simulink model "LR_Traject_Sim"  (R2017b)
settings: Solver=ode4  StartTime=0  StopTime=100  FixedStep=0.05  RelTol=1e-7
model workspace (MAT data in the model file):
  Object = Simulink.LookupTable
  Object.Table = Simulink.lookuptable.Table
  Object.Table.Dimensions = [0 0]
  Object.Table.DataType = 'auto'
  Object.Table.FieldName = 'Table'
  Object.Breakpoints = Simulink.lookuptable.Breakpoint
  Object.Breakpoints.TunableSizeName = 'N1'
  Object.Breakpoints.Dimensions = [0 0]
  Object.Breakpoints.DataType = 'auto'
  Object.Breakpoints.FieldName = 'BP1'
  Object.SupportTunableSize = 0
  Object.StructTypeInfo = Simulink.lookuptable.StructTypeInfo
  Object.StructTypeInfo.DataScope = 'Auto'
undefined symbols (not defined in the file or in its folder): Conditions, Eng, Roc
settings Model: Creator=adamb  LastModifiedBy=dc0069
settings SolverCC: ZeroCrossAlgorithm=Adaptive
settings DataIOCC: SaveFormat=StructureWithTime
settings OptimizationCC: LifeSpan=inf
settings DebuggingCC: AlgebraicLoopMsg=none  ArtificialAlgebraicLoopMsg=none  SFExecutionAtInitializationDiag=none
settings HardwareCC: ProdBitPerSizeT=32  ProdBitPerPtrDiffT=32  ProdWordSize=32  ProdHWDeviceType=Specified
settings CodeAppCC: StateflowObjectComments=on
settings SimscapeCC: SimscapeNormalizeSystem=off
settings ConfigurationSet: Description=SimMechanics 2G

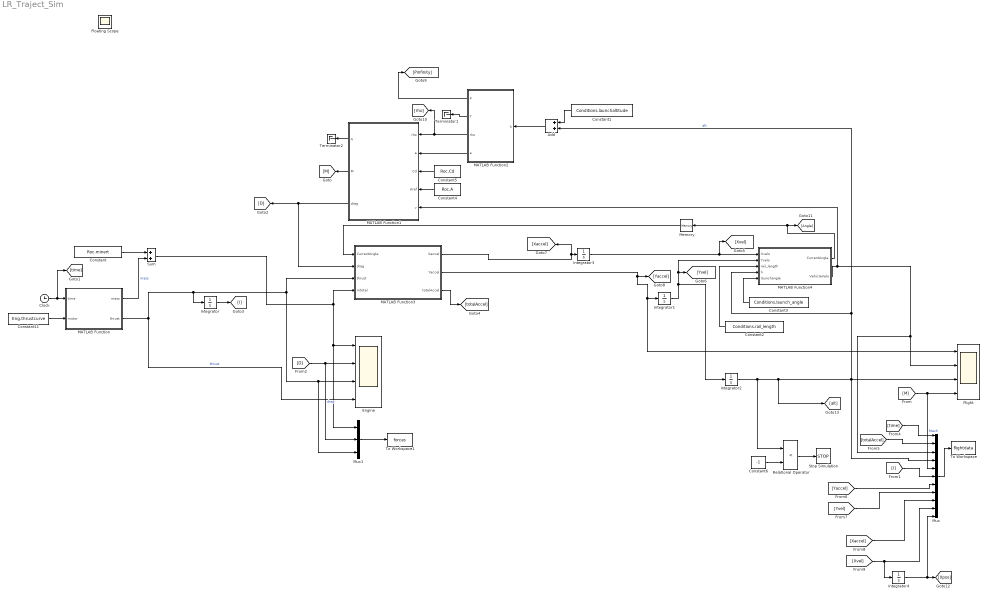
== system LR_Traject_Sim ==
  Add : Sum
  Clock : Clock
  Constant : Constant  Value=Roc.minert
  Constant1 : Constant  Value=Conditions.launchaltitude
  Constant11 : Constant  Value=Eng.thrustcurve
  Constant2 : Constant  Value=Conditions.rail_length
  Constant3 : Constant  Value=Conditions.launch_angle
  Constant4 : Constant  Value=Roc.A
  Constant5 : Constant  Value=Roc.Cd  VectorParams1D=off
  Constant6 : Constant  Value=-1
  Engine : Scope  NumInputPorts=4
  Flight : Scope  NumInputPorts=4
  Integrator{,1..4} (5 alike) : Integrator
  MATLAB Function : MATLAB Function  TreatAsAtomicUnit=on
  MATLAB Function1 : MATLAB Function  TreatAsAtomicUnit=on
  MATLAB Function2 : MATLAB Function  TreatAsAtomicUnit=on
  MATLAB Function3 : MATLAB Function  TreatAsAtomicUnit=on
  MATLAB Function4 : MATLAB Function  TreatAsAtomicUnit=on
  Memory : Memory
  Mux : Mux  Inputs=11
  Mux1 : Mux  Inputs=3
  Relational Operator : RelationalOperator  Operator=<  OutDataTypeStr=boolean  RndMeth=Nearest
  Stop Simulation : Stop
  Sum : Sum
  Terminator1 : Terminator
  Terminator2 : Terminator
  To Workspace : ToWorkspace  VariableName=flightdata  SampleTime=-1
  To Workspace1 : ToWorkspace  VariableName=forces  SampleTime=-1
  Floating Scope : Scope
  wires:
  MATLAB Function/1(mass) -> Sum/2  "mass"
  MATLAB Function/2(thrust) -> Engine/4, Mux1/3, Engine/3, MATLAB Function3/3(thrust), Integrator/1  "thrust"
  Integrator1/1 -> Integrator2/1, [Yvel], MATLAB Function4/2(Yvelo)
  Integrator2/1 -> Relational Operator/1, Add/2, MATLAB Function4/4(h), Flight/3, Mux/4, [alt]  "alt"
  Constant4/1 -> MATLAB Function1/4(Aref)
  Constant5/1 -> MATLAB Function1/3(Cd)
  MATLAB Function1/2(M) -> [M]
  [M] -> Mux/5, Flight/4  "Mach"
  MATLAB Function1/3(drag) -> [D], MATLAB Function3/2(drag)
  Relational Operator/1 -> Stop Simulation/1
  Constant6/1 -> Relational Operator/2
  MATLAB Function2/4(a) -> MATLAB Function1/2(a)
  MATLAB Function2/3(rho) -> [rho], MATLAB Function1/1(rho)
  Mux/1 -> To Workspace/1
  MATLAB Function2/2(T) -> Terminator1/1
  [D] -> Mux1/2, Engine/2  "drag"
  Mux1/1 -> To Workspace1/1
  MATLAB Function1/1(q) -> Terminator2/1
  MATLAB Function2/1(P) -> [Pinfinity]
  Clock/1 -> MATLAB Function/1(time), [time]
  [time] -> Mux/1
  MATLAB Function3/2(Yaccel) -> Flight/1, Integrator1/1, [Yaccel]
  Integrator3/1 -> [Xvel], MATLAB Function4/1(Xvelo)
  MATLAB Function4/2(VehicleVelo) -> MATLAB Function1/5(v), Flight/2, Mux/3
  Integrator/1 -> [I]
  [I] -> Mux/6
  Add/1 -> MATLAB Function2/1(h)
  Constant1/1 -> Add/1
  MATLAB Function4/1(CurrentAngle) -> [Angle], Memory/1
  Constant2/1 -> MATLAB Function4/3(rail_length)
  Constant3/1 -> MATLAB Function4/5(launchangle)
  Memory/1 -> MATLAB Function3/1(CurrentAngle)
  [totalAccel] -> Mux/2
  [Xaccel] -> Mux/9
  [Xvel] -> Integrator4/1, Mux/10
  [Yvel] -> Mux/8
  [Yaccel] -> Mux/7
  Integrator4/1 -> [Xpos], Mux/11
  MATLAB Function3/1(Xaccel) -> [Xaccel], Integrator3/1
  MATLAB Function3/3(totalAccel) -> [totalAccel]
  Constant/1 -> Sum/1
  Sum/1 -> Mux1/1, Engine/1, MATLAB Function3/4(mtotal)
  Constant11/1 -> MATLAB Function/2(motor)

== matlab function LR_Traject_Sim/MATLAB Function1 ==
  data: rho input; a input; q output; M output; Cd input; Aref input; v input; drag output
function [q,M,drag] = AeroComputation(rho,a,Cd,Aref,v)

M = abs(v/a); % Mach #
q = 0.5*rho*abs(v)*v; % qbar, Dynamic Pressure

A = Aref(1);
CdM = interp1(Cd(1,:),Cd(2,:),M); % Interpolates the Cd based on M

drag = q*A*CdM;

%fprintf('Velocity is %f, drag is %f, rho is %f, a is %f, Cdm is %f\n', v, drag, rho, a, CdM);


end

== matlab function LR_Traject_Sim/MATLAB Function2 ==
  data: h input; P output; T output; rho output; a output
function [P,T,rho,a] = AtmosParams(h)

[P,rho,T,a] = StdAtmos(h);

end

== matlab function LR_Traject_Sim/MATLAB Function3 ==
  data: CurrentAngle input; drag input; Xaccel output; thrust input; mtotal input; Yaccel output; totalAccel output
function [Xaccel, Yaccel, totalAccel] = AccelerationComponents(CurrentAngle, drag, thrust, mtotal)

%Direction of current velocity vector equals Current Angle
%Thrust and drag are assumed along the axis of the velocity
%Gravity is constant 9.81m/s^2 along the y-axis

%Constants
AccelGravity = -9.81;

AccelDrag = drag/mtotal; %Acceleration caused by drag
AccelThrust = thrust/mtotal; %Acceleration caused by Thrust
AccelRocket = AccelThrust-AccelDrag; %Acceleration of Rocket
Yaccel = AccelRocket * cos(CurrentAngle) + AccelGravity; %Acceleration of Rocket in Y Direction
Xaccel = AccelRocket * sin(CurrentAngle); %Acceleration of rocket in x direction
totalAccel = sqrt(Xaccel^2 + Yaccel^2);

== matlab function LR_Traject_Sim/MATLAB Function4 ==
  data: Xvelo input; CurrentAngle output; Yvelo input; rail_length input; VehicleVelo output; h input; launchangle input
function [CurrentAngle, VehicleVelo]  = CurrentAngle(Xvelo,Yvelo, rail_length, h, launchangle)

%This function's main purpose is to calculate current vehicle angle without
%using two simulink math blocks vs one function block.

%Pretty cool huh?

CurrentAngle = atan(Xvelo/Yvelo);
VehicleVelo = sqrt(Xvelo^2+Yvelo^2);

if h < rail_length
    CurrentAngle = launchangle;
end

== matlab function LR_Traject_Sim/MATLAB Function ==
  data: mass output; time input; thrust output; motor input
function [mass, thrust] = solidThrust(time, motor)

data = motor.thrustcurve;
% If t is after the end of the data, thrust is 0
if t >= data(end, 1)
    thrust = 0;
else

    % Find the data point before this time
    for before = 1:(length(data) - 1)
        if data(before + 1, 1) > t
            break;
        end
    end
    % And the data point after this time
    after = before + 1;
    % Calculate thrust through linear interpolation between the thrust before
    % and the thrust after the target time
    thrust = data(before, 2) + (t - data(before, 1)) * ...
        (data(after, 2) - data(before, 2)) / ...
        (data(after, 1) - data(before, 1));
end

if time >= motor.burntime
    mass = motor.mfinal;
else
    mass = motor.minitial - (time / motor.burntime) * (motor.minitial - motor.mfinal);
end
end
